simulink model "SafetyCriticalLQR"  (R2020b)
settings: Solver=VariableStepAuto  StartTime=0.0  StopTime=tf_upperbound  RelTol=1e-7  AbsTol=1e-7
PreLoadFcn:
  | SafetyCriticalLQRParams
values from neighbouring files (symbols this model uses):
  A = [0  1; 0  0]    [RCBF_LinProgTrick_WorstCaseTrajectory_90Percent.mat]    (also in RCBF_LinProgTrick_WorstCaseTrajectory_DifferentBeta.mat)
  B = [0 1]    [RCBF_LinProgTrick_WorstCaseTrajectory_90Percent.mat]    (also in RCBF_LinProgTrick_WorstCaseTrajectory_DifferentBeta.mat)
  beta = 0.8    [RCBF_LinProgTrick_WorstCaseTrajectory.m]    (also in RCBF_LinProgTrick_WorstCaseTrajectory_90Percent.mat = 0.9; RCBF_LinProgTrick_WorstCaseTrajectory_DifferentBeta.mat = 0.9)
  C = [1  0; 0  1]    [RCBF_LinProgTrick_WorstCaseTrajectory_90Percent.mat]    (also in RCBF_LinProgTrick_WorstCaseTrajectory_DifferentBeta.mat)
  cT = [10 -5]    [RCBF_LinProgTrick_WorstCaseTrajectory_90Percent.mat]    (also in RCBF_LinProgTrick_WorstCaseTrajectory_DifferentBeta.mat)
  D = [0 0]    [RCBF_LinProgTrick_WorstCaseTrajectory_90Percent.mat]    (also in RCBF_LinProgTrick_WorstCaseTrajectory_DifferentBeta.mat)
  eta = 2    [RCBF_LinProgTrick_WorstCaseTrajectory_90Percent.mat]    (also in RCBF_LinProgTrick_WorstCaseTrajectory_DifferentBeta.mat)
  filterCase = 4    [RCBF_LinProgTrick_WorstCaseTrajectory.m]    (also in RCBF_LinProgTrick_WorstCaseTrajectory_90Percent.mat; RCBF_LinProgTrick_WorstCaseTrajectory_DifferentBeta.mat)
  gamma = 1    [RCBF_LinProgTrick_WorstCaseTrajectory_90Percent.mat]    (also in RCBF_LinProgTrick_WorstCaseTrajectory_DifferentBeta.mat)
  K = [0.316227766017 0.855836159574]    [RCBF_LinProgTrick_WorstCaseTrajectory_90Percent.mat]    (also in RCBF_LinProgTrick_WorstCaseTrajectory_DifferentBeta.mat)
  lambda = 1    [RCBF_LinProgTrick_WorstCaseTrajectory_DifferentBeta.mat]
  P = [1.35319578409  1.58113883008; 1.58113883008  4.27918079787]    [RCBF_LinProgTrick_WorstCaseTrajectory_90Percent.mat]    (also in RCBF_LinProgTrick_WorstCaseTrajectory_DifferentBeta.mat)
  Ref = [0 0]    [RCBF_LinProgTrick_WorstCaseTrajectory_90Percent.mat]    (also in RCBF_LinProgTrick_WorstCaseTrajectory_DifferentBeta.mat)
  rT = 4    [RCBF_LinProgTrick_WorstCaseTrajectory_90Percent.mat]    (also in RCBF_LinProgTrick_WorstCaseTrajectory_DifferentBeta.mat)
  x0 = [10 10]    [RCBF_LinProgTrick_WorstCaseTrajectory_90Percent.mat]    (also in RCBF_LinProgTrick_WorstCaseTrajectory_DifferentBeta.mat)
libraries: simulink x2
settings Model: Creator=Jyot Buch  LastModifiedBy=Jyot Buch

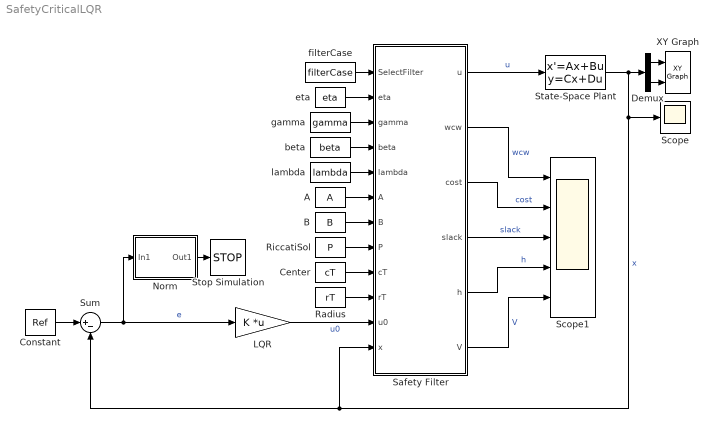
== system SafetyCriticalLQR ==
  A : Constant  Value=A
  B : Constant  Value=B
  Center : Constant  Value=cT
  Constant : Constant  Value=Ref
  Demux : Demux  Outputs=2
  LQR : Gain  Gain=K  Multiplication=Matrix(K*u) (u vector)
  Norm : Subsystem
  Radius : Constant  Value=rT
  RiccatiSol : Constant  Value=P
  Safety Filter : MATLAB Function  TreatAsAtomicUnit=on
  Scope : Scope
  Scope1 : Scope  NumInputPorts=5
  State-Space Plant : StateSpace  A=A  B=B  C=C  D=D  InitialCondition=x0
  Stop Simulation : Stop
  Sum : Sum  Inputs=|+-
  XY Graph : simulink/Sinks/XY Graph  xmin=-20  xmax=20  ymin=-15  ymax=15  st=-1
  beta : Constant  Value=beta
  eta : Constant  Value=eta
  filterCase : Constant  Value=filterCase
  gamma : Constant  Value=gamma
  lambda : Constant  Value=lambda
  wires:
  State-Space Plant/1 -> Safety Filter/12(x), Sum/2, Scope/1, Demux/1  "x"
  Constant/1 -> Sum/1
  Sum/1 -> LQR/1, Norm/1(In1)  "e"
  LQR/1 -> Safety Filter/11(u0)  "u0"
  Safety Filter/1(u) -> State-Space Plant/1  "u"
  Radius/1 -> Safety Filter/10(rT)
  Demux/2 -> XY Graph/2
  Demux/1 -> XY Graph/1
  filterCase/1 -> Safety Filter/1(SelectFilter)
  Center/1 -> Safety Filter/9(cT)
  RiccatiSol/1 -> Safety Filter/8(P)
  Safety Filter/5(h) -> Scope1/4  "h"
  Safety Filter/6(V) -> Scope1/5  "V"
  Norm/1(Out1) -> Stop Simulation/1
  eta/1 -> Safety Filter/2(eta)
  gamma/1 -> Safety Filter/3(gamma)
  Safety Filter/4(slack) -> Scope1/3  "slack"
  A/1 -> Safety Filter/6(A)
  B/1 -> Safety Filter/7(B)
  beta/1 -> Safety Filter/4(beta)
  Safety Filter/2(wcw) -> Scope1/1  "wcw"
  lambda/1 -> Safety Filter/5(lambda)
  Safety Filter/3(cost) -> Scope1/2  "cost"

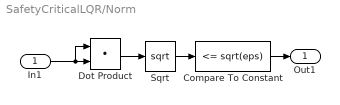
== system SafetyCriticalLQR/Norm ==
  In1 : Inport
  Compare To Constant : simulink/Logic and Bit Operations/Compare To Constant  relop=<=  const=sqrt(eps)  OutDataTypeStr=boolean
  Dot Product : DotProduct  InputSameDT=on  OutDataTypeStr=Inherit: Inherit via internal rule
  Sqrt : Sqrt  SaturateOnIntegerOverflow=on
  Out1 : Outport
  wires:
  In1/1 -> Dot Product/1, Dot Product/2
  Dot Product/1 -> Sqrt/1
  Sqrt/1 -> Compare To Constant/1
  Compare To Constant/1 -> Out1/1

== matlab function SafetyCriticalLQR/Safety Filter ==
  data: u output; wcw output; cost output; SelectFilter input; eta input; gamma input; beta input; lambda input; A input; B input; P input; cT input; rT input; u0 input; slack output; x input; h output; V output
function [u,wcw,cost,slack,h,V] = fcn(SelectFilter,eta,gamma,beta,lambda,A,B,P,cT,rT,u0,x)
%% FCN
% Compute h and V
h = (x(1)-cT(1))^2 + (x(2)-cT(2))^2 - rT^2;
V = x'*P*x;
slack = 0;
cost = 0;

% Select filter based on the specified case
switch SelectFilter
    case 1
        % Nominal LQR
        u = u0;
        
    case 2
        % CBF Only
        [u,cost] = CBFQP(eta,h,cT,u0,x);
        
    case 3
        % CLF-CBF
        [u,cost,slack] = CLFCBFQP(eta,gamma,h,V,A,B,P,cT,u0,x);
        
    case 4
        % Robust CBF with LinProgTick
        [u,cost] = RobustCBFQPLinProgTick(eta,beta,h,cT,u0,x);
        
    case 5
        % Robust CBF with QCQP
        [u,cost] = RobustCBFQCQP(eta,beta,lambda,h,cT,u0,x);
        
    otherwise
        % Openloop
        u = u0*0;
end

% Worst-case uncertainty
wcw = -beta*abs(u)*sign(x(2)-cT(2));
end

%% CBFQP
function [u,cost] = CBFQP(eta,h,cT,u0,x)
% Inequality Safety Constraints for QP
% Aineq'*u <= bineq
Aineq = -2*(x(2)-cT(2));
bineq = 2*(x(1)-cT(1))*x(2) + eta*h;

% Solve QP
SolveQPCase = 1;
switch SolveQPCase
    case 1
        % Numerical Solution
        H = 1;
        f = -u0;
        opt = optimoptions('quadprog','Algorithm','active-set','Display','off');
        [u,cost] = quadprog(H,f,Aineq,bineq,[],[],[],[],u0,opt);
        cost = cost + 0.5*(u0'*u0);
        
    case 2
        % Explicit Solution
        rho = -bineq+Aineq*u0;
        if rho<=0
            zopt = 0;
        else
            zopt = -rho*Aineq/Aineq^2;
        end
        u = zopt+u0;
        cost = 0.5*(zopt'*zopt);
end
end

%% CLFCBFQP
function [u,cost,slack] = CLFCBFQP(eta,gamma,h,V,A,B,P,cT,u0,x)
% Slack variable penalty
m = 1;

% Inequality Constraints for QP
% Safety: hdot >= -alpha*h
Aineq1 = [-2*(x(2)-cT(2)) 0];
bineq1 = 2*(x(1)-cT(1))*x(2) + eta*h;

% Stability: Vdot <= -beta*V
Aineq2 = [2*x'*P*B -1];
bineq2 = -x'*(A'*P + P*A)*x - gamma*V;

% Aineq'*[u;delta] <= bineq
Aineq = [Aineq1; Aineq2];
bineq = [bineq1; bineq2];

% Solve QP
H = diag([1, m]);
opt = optimoptions('quadprog','Algorithm','active-set','Display','off');
[sol,cost] = quadprog(H,[],Aineq,bineq,[],[],[],[],[u0;0],opt);

% Read outputs
u = sol(1);
slack = sol(2);
end

%% RobustCBFQPLinProgTick
function [u,cost] = RobustCBFQPLinProgTick(eta,beta,h,cT,u0,x)
% Inequality Constraints for QP
% Aineq'*u <= bineq
p = x(2)-cT(2);
Aineq = [-2*p*(1 - sign(p)*beta) +2*p*(sign(p)*beta + 1); -1 0;0 -1];
bineq = [2*(x(1)-cT(1))*x(2) + eta*h; 0; 0];

% Solve QP
H = [1 -1;-1 1];
f = [-u0 +u0];
opt = optimoptions('quadprog','Algorithm','active-set','Display','off');
[uStar,cost] = quadprog(H,f,Aineq,bineq,[],[],[],[],[u0;u0]*0,opt);
cost = cost + 0.5*(u0'*u0);

% up and un
up = uStar(1);
un = uStar(2);

% Output
u = up - un;
end

%% RobustCBFQCQP
function [u,cost] = RobustCBFQCQP(eta,beta,lambda,h,cT,u0,x)
% Objective
objective = @(u) 0.5*(u-u0)'*(u-u0);

% Constraints
constraint = @NestedFunction;

% NestedFunction
    function [c,ceq] = NestedFunction(u)
        c = -eta*h - 2*(x(1)-cT(1))*x(2) - 2*(x(2)-cT(2))*u + lambda*beta^2*u^2 + (1/lambda^2)*(x(2)-cT(2))^2;
        ceq = 0;
    end

% Solve optimization problem
options = optimoptions('fmincon','Display','off','Algorithm','sqp');
[u,cost,exitflag,output]  = fmincon(objective,u0,[],[],[],[],[],[],constraint,options); %#ok<ASGLU>
end
